simulink model "ArtPanRev1"  (R2019b)
settings: Solver=VariableStepAuto  StartTime=0.0  StopTime=10.0  RelTol=1e-3
values from neighbouring files (symbols this model uses):
  th2 = 50    [AP_TimeDelay.m]    (also in SmithControl.m; TimeDelayParameters.m; positivity_matrix.m; rscale.m)
  th3 = 60    [AP_TimeDelay.m]    (also in SmithControl.m; TimeDelayParameters.m = 70; positivity_matrix.m; rscale.m)
  th4 = 5    [AP_TimeDelay.m]    (also in SmithControl.m; TimeDelayParameters.m = 2.7; positivity_matrix.m; rscale.m)
  th5 = 20    [AP_TimeDelay.m]    (also in SmithControl.m; TimeDelayParameters.m = 22; positivity_matrix.m; rscale.m)
undefined symbols (not defined in the file or in its folder): Gr, k_aw, ki, kp
settings Model: Creator=akshita_jain  LastModifiedBy=akshita_jain

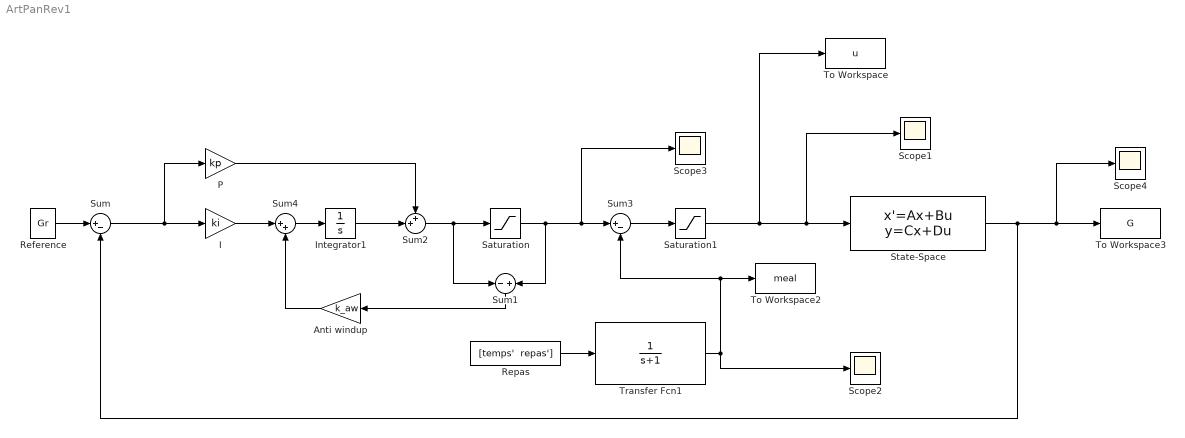
== system ArtPanRev1 ==
  "Anti windup " : Gain  Gain=k_aw
  I : Gain  Gain=ki
  Integrator1 : Integrator  InitialCondition=0.001
  P : Gain  Gain=kp
  Reference : Constant  Value=Gr
  Repas : FromWorkspace  VariableName="[temps'  repas']"  SampleTime=0
  Saturation : Saturate  UpperLimit=2  LowerLimit=0
  Saturation1 : Saturate  UpperLimit=inf  LowerLimit=0
  Scope{1..4} (4 alike) : Scope
  State-Space : StateSpace  A=[0 -th2 0 th4 0; 0 -1/th3 1/th3 0 0; 0 0 -1/th3 0 0; 0 0 0 -1/th5 1/th5; 0 0 0 0 -1/th5]  B=[0 0; 0 0; 1/th3 0; 0 0; 0 1/th5]  C=[1 0 0 0 0]  D=[0 0]  InitialCondition=0
  Sum : Sum  Inputs=|+-
  Sum1 : Sum  Inputs=-+
  Sum2 : Sum  Inputs=++|
  Sum3 : Sum  Inputs=|+-
  Sum4 : Sum  Inputs=|++
  To Workspace : ToWorkspace  VariableName=u  SampleTime=-1
  To Workspace2 : ToWorkspace  VariableName=meal  SampleTime=-1
  To Workspace3 : ToWorkspace  VariableName=G  SampleTime=-1
  Transfer Fcn1 : TransferFcn  Numerator=[0 0 1]  Denominator=[1 1]
  wires:
  P/1 -> Sum2/1
  Sum2/1 -> Saturation/1, Sum1/1
  Repas/1 -> Transfer Fcn1/1
  Sum4/1 -> Integrator1/1
  I/1 -> Sum4/1
  Sum/1 -> I/1, P/1
  Sum3/1 -> Saturation1/1
  Integrator1/1 -> Sum2/2
  "Anti windup "/1 -> Sum4/2
  Saturation/1 -> Scope3/1, Sum3/1, Sum1/2
  Transfer Fcn1/1 -> Sum3/2, To Workspace2/1, Scope2/1
  Reference/1 -> Sum/1
  State-Space/1 -> Sum/2, To Workspace3/1, Scope4/1
  Sum1/1 -> "Anti windup "/1
  Saturation1/1 -> Scope1/1, State-Space/1, To Workspace/1
